simulink model "FingerEAERCtrl"  (R2012b)
settings: Solver=ode3  StartTime=0.0  StopTime=inf  FixedStep=.001  RelTol=1e-3
PreLoadFcn:
  | settupFilter;
InitFcn:
  | settupFilter;
values from neighbouring files (symbols this model uses):
  x0low = (eye(size(Alow))-Alow)\Blow*0    [settupFilter.m]
undefined symbols (not defined in the file or in its folder): Alow, Blow, Clow, Dlow
libraries: xpcnilib x4, xpclib x4, simulink x2
(part 2 of 2)

== system FingerEAERCtrl/trajectory calculator/mode 4: sub init no return/rt minimum jerk trajectory1/params buffer1 ==
  pDes_ : Inport
  tHit_ : Inport  Port=2
  maxDur : Inport  Port=3
  t : Inport  Port=4
  Trigger : TriggerPort  PortDimensions=1
  Memory : Memory  InheritSampleTime=on
  Memory1 : Memory  InheritSampleTime=on
  buffer the trajectory params : MATLAB Function  TreatAsAtomicUnit=on
  pDes : Outport
  tHit : Outport  Port=2
  dur : Outport  Port=3
  wires:
  pDes_/1 -> buffer the trajectory params/1(pDes_)
  buffer the trajectory params/1(pDes) -> pDes/1
  buffer the trajectory params/2(tHit) -> Memory/1, tHit/1
  tHit_/1 -> buffer the trajectory params/2(tHit_)
  t/1 -> buffer the trajectory params/4(t)
  maxDur/1 -> buffer the trajectory params/3(maxDur)
  buffer the trajectory params/3(dur) -> Memory1/1, dur/1
  Memory/1 -> buffer the trajectory params/5(lastHit)
  Memory1/1 -> buffer the trajectory params/6(lastDur)

== system FingerEAERCtrl/trajectory calculator/mode 4: sub init no return/rt minimum jerk trajectory1/saveTrialStartTime ==
  t : Inport
  Trigger : TriggerPort  PortDimensions=1
  save the trial start time : MATLAB Function  TreatAsAtomicUnit=on
  trialStartTime : Outport
  wires:
  t/1 -> save the trial start time/1(t)
  save the trial start time/1(trialStartTime) -> trialStartTime/1

== system FingerEAERCtrl/trajectory calculator/mode 4: sub init no return/rt minimum jerk trajectory1/timeToTrigger ==
  note: This block (triggered by passing the force threshold / success in the movement initiation)
      | checks to make sure that it wasn't a subsequent trigger, and if it wasn't, passes the time
      | from the trial start to the time of the trigger event (time to meet the force threshold) as feedback
  t : Inport
  trialStart : Inport  Port=2
  Trigger : TriggerPort  PortDimensions=1
  Memory : Memory  InheritSampleTime=on
  Memory1 : Memory  InheritSampleTime=on
  save the trigger time : MATLAB Function  TreatAsAtomicUnit=on
  triggerTime : Outport
  wires:
  t/1 -> save the trigger time/2(t)
  trialStart/1 -> save the trigger time/3(trialStart)
  save the trigger time/2(lastStartT) -> Memory/1
  Memory/1 -> save the trigger time/4(lastTrialStart)
  save the trigger time/1(triggerTime) -> Memory1/1, triggerTime/1
  Memory1/1 -> save the trigger time/1(lastTriggerTime)

== system FingerEAERCtrl/trajectory calculator/mode 4: sub init no return/rt minimum jerk trajectory2/detect new trajectory ==
  note: detects when tDes is changed, and trips the trigger
  tDes : Inport
  MATLAB Function1 : MATLAB Function  TreatAsAtomicUnit=on
  Memory2 : Memory
  change : Outport
  wires:
  tDes/1 -> MATLAB Function1/1(tDes)
  MATLAB Function1/1(change) -> change/1
  MATLAB Function1/2(tDesOut) -> Memory2/1
  Memory2/1 -> MATLAB Function1/2(tDesLast)

== system FingerEAERCtrl/trajectory calculator/mode 4: sub init no return/rt minimum jerk trajectory2/force buffer ==
  force_ : Inport
  Trigger : TriggerPort  PortDimensions=1
  buffer the initial force value : MATLAB Function  TreatAsAtomicUnit=on
  force : Outport
  wires:
  force_/1 -> buffer the initial force value/1(force_)
  buffer the initial force value/1(force) -> force/1

== system FingerEAERCtrl/trajectory calculator/mode 4: sub init no return/rt minimum jerk trajectory2/params buffer1 ==
  pDes_ : Inport
  tHit_ : Inport  Port=2
  maxDur : Inport  Port=3
  t : Inport  Port=4
  Trigger : TriggerPort  PortDimensions=1
  Memory : Memory  InheritSampleTime=on
  Memory1 : Memory  InheritSampleTime=on
  buffer the trajectory params : MATLAB Function  TreatAsAtomicUnit=on
  pDes : Outport
  tHit : Outport  Port=2
  dur : Outport  Port=3
  wires:
  pDes_/1 -> buffer the trajectory params/1(pDes_)
  buffer the trajectory params/1(pDes) -> pDes/1
  buffer the trajectory params/2(tHit) -> Memory/1, tHit/1
  tHit_/1 -> buffer the trajectory params/2(tHit_)
  t/1 -> buffer the trajectory params/4(t)
  maxDur/1 -> buffer the trajectory params/3(maxDur)
  buffer the trajectory params/3(dur) -> Memory1/1, dur/1
  Memory/1 -> buffer the trajectory params/5(lastHit)
  Memory1/1 -> buffer the trajectory params/6(lastDur)

== system FingerEAERCtrl/trajectory calculator/mode 4: sub init no return/rt minimum jerk trajectory2/saveTrialStartTime ==
  t : Inport
  Trigger : TriggerPort  PortDimensions=1
  save the trial start time : MATLAB Function  TreatAsAtomicUnit=on
  trialStartTime : Outport
  wires:
  t/1 -> save the trial start time/1(t)
  save the trial start time/1(trialStartTime) -> trialStartTime/1

== system FingerEAERCtrl/trajectory calculator/mode 4: sub init no return/rt minimum jerk trajectory2/timeToTrigger ==
  note: This block (triggered by passing the force threshold / success in the movement initiation)
      | checks to make sure that it wasn't a subsequent trigger, and if it wasn't, passes the time
      | from the trial start to the time of the trigger event (time to meet the force threshold) as feedback
  t : Inport
  trialStart : Inport  Port=2
  Trigger : TriggerPort  PortDimensions=1
  Memory : Memory  InheritSampleTime=on
  Memory1 : Memory  InheritSampleTime=on
  save the trigger time : MATLAB Function  TreatAsAtomicUnit=on
  triggerTime : Outport
  wires:
  t/1 -> save the trigger time/2(t)
  trialStart/1 -> save the trigger time/3(trialStart)
  save the trigger time/2(lastStartT) -> Memory/1
  Memory/1 -> save the trigger time/4(lastTrialStart)
  save the trigger time/1(triggerTime) -> Memory1/1, triggerTime/1
  Memory1/1 -> save the trigger time/1(lastTriggerTime)

== matlab function FingerEAERCtrl/trajectory calculator/mode 1: sub-init/rt minimum jerk trajectory calc/detect movement onset ==
  data: pos input; vel input; V_THRESH input; tDes input; update output; t input; pTraj input; maxDur input
% this function will detect when the subject startes to move. As soon as
% the subject's velocity reaches a certain threshold, get the distance to
% the target and the start time
function update = checkUpdate(pos, vel, V_THRESH, tDes, t, pTraj, maxDur)
%#codegen
update = 0;
if ((vel > V_THRESH) && (t < tDes) && (pTraj == 0))
    %% add another condition to make sure that the robot does not try to move super fast
    if ((abs(tDes - t) > .15) && (abs(tDes - t) < maxDur))
        update = 1;
    end    
end

== matlab function FingerEAERCtrl/controller/controller ==
  data: stateDes input; Forces output; state input; Kp input; Kd input
function Forces = pdCtrl(stateDes, state, Kp, Kd)
%#codegen
pDes = [stateDes(1); stateDes(4)];
vDes = [stateDes(2); stateDes(5)];

pos = [state(1); state(3)];
vel = [state(2); state(4)];

error = pDes - pos;
errorDot = vDes - vel;

Forces = error.*Kp + errorDot.*Kd;

== matlab function FingerEAERCtrl/trajectory calculator/mode 1: sub-init/rt minimum jerk trajectory calc/params buffer/buffer the trajectory params ==
  data: pDes output; tHit output; pDes_ input; tHit_ input; t input; dur output
function [pDes, tHit, dur] = bufferParams(pDes_, tHit_, t)
%#codegen
pDes = pDes_;
tHit = tHit_;
dur = tHit_ - t;
% Ro = abs(pDes - pos)
% to = t
% tr = tDes - to

== matlab function FingerEAERCtrl/trajectory calculator/mode 1: sub-init/rt minimum jerk trajectory calc/MATLAB Function ==
  data: Pd input; th input; dur input; des output; t input
% th is the hit time
% Pd id the final destination
% t is the current time
% dur is the duration 
function des = trajCalc(Pd, th, dur, t)
%#codegen
startT = th - dur;  % number of miliseconds until the hit time
returnT = th + dur;  % return time

if t > startT && t<=th
T=t-(startT);
des=[(10*Pd*T^3)/dur^3 - (15*Pd*T^4)/dur^4 + (6*Pd*T^5)/dur^5;...
(30*Pd*T^2)/dur^3 - (60*Pd*T^3)/dur^4 + (30*Pd*T^4)/dur^5;...
(120*Pd*T^3)/dur^5 - (180*Pd*T^2)/dur^4 + (60*Pd*T)/dur^3];
elseif th<t && t<returnT
T=t-th;
des=[Pd - (10*Pd*T^3)/dur^3 + (15*Pd*T^4)/dur^4 - (6*Pd*T^5)/dur^5;...
(60*Pd*T^3)/dur^4 - (30*Pd*T^2)/dur^3 - (30*Pd*T^4)/dur^5;...
(180*Pd*T^2)/dur^4 - (120*Pd*T^3)/dur^5 - (60*Pd*T)/dur^3];
else
des=[0;0;0];
end

== matlab function FingerEAERCtrl/trajectory calculator/mode 3: auto init no return/rt minimum jerk trajectory/MATLAB Function ==
  data: Pd input; th input; dur input; des output; t input; Phold_ input; Phold output; state_ input; state output
% th is the hit time
% Pd id the final destination
% t is the current time
% dur is the duration 
function [des, Phold, state] = trajCalc(Pd, th, dur, t, Phold_, state_)
startT = th - dur;  % number of miliseconds until the hit time

Pr = Pd - Phold_;
Phold = Phold_;
state = state_;
switch state_
    case 0
        des = [Phold_; 0; 0];
        if (t > startT); state = 1; end
    case 1
        T=t-(startT);
        des=[(10*Pr*T^3)/dur^3 - (15*Pr*T^4)/dur^4 + (6*Pr*T^5)/dur^5 + Phold_;...
        (30*Pr*T^2)/dur^3 - (60*Pr*T^3)/dur^4 + (30*Pr*T^4)/dur^5;...
        (120*Pr*T^3)/dur^5 - (180*Pr*T^2)/dur^4 + (60*Pr*T)/dur^3];
        if (t > th); state = 2; end
    case 2
        Phold = Pd;
        des = [Pd; 0; 0];
        state = 3;
    case 3
        des = [Phold_; 0; 0];
        if (t < startT); state = 0; end
    otherwise
        state = 0;
        Phold = 0;
        des = [Phold_; 0; 0];
end

== matlab function FingerEAERCtrl/trajectory calculator/mode 3: auto init no return/rt minimum jerk trajectory/detect change/MATLAB Function1 ==
  data: pDes input; change output; pDes_ input
function change = detectChange(pDes, pDes_)
%#codegen
change = 0
diffS = pDes - pDes_;
if (diffS > 0) && (pDes_ == 0)
    change = 1;
end

== matlab function FingerEAERCtrl/trajectory calculator/mode 3: auto init no return/rt minimum jerk trajectory/params buffer/buffer the trajectory params ==
  data: pDes output; tHit output; pDes_ input; tHit_ input
function [pDes, tHit] = bufferParams(pDes_, tHit_)
%#codegen
pDes = pDes_;
tHit = tHit_;
% Ro = abs(pDes - pos)
% to = t
% tr = tDes - to

== matlab function FingerEAERCtrl/controller/gain transition/gainramp ==
  data: val output; tr input; valD input; state1 output; state input
% state contains [valD_,val_,Ro_,t_]
function [val,state1] = fcn(tr,valD,state)
%#eml

% first we need to check if they have changed the desired Value
if ~ (valD == state(1))
    state(1) = valD;
    state(4) = 0;
    state(3) = state(1) - state(2);
end

t = state(4);
Ro = state(3);

if ((t <= tr) && (tr~=0))
    Rd = Ro - Ro*(10*(t)^3/(tr)^3 - 15*(t)^4/(tr)^4 + 6*(t)^5/(tr)^5);
else
    Rd = 0;
end

val = state(1) - Rd;
state(2) = val;
state(4) = t + .001;
state1 = state;

== matlab function FingerEAERCtrl/Robot/get offsets/MATLAB Function ==
  data: enc1_ input; encoder1 output; enc2_ input; time input; summedVals_ input; nSamples_ input; encoder2 output; summedVals output; nSamples output
%% remove the position offset that comes from using the encoders for
% feedback
%%
function [encoder1, encoder2, summedVals, nSamples] = getOffset(enc1_, enc2_, time, summedVals_, nSamples_)
%#codegen
summedVals = summedVals_;
if (time > 2) && (time < 3)
    summedVals(1) = summedVals_(1) + enc1_;
    summedVals(2) = summedVals_(2) + enc2_;
    nSamples = nSamples_ + 1;
    encoder1 = 0;
    encoder2 = 0;
elseif (time >=3)
    summedVals = summedVals_;
    nSamples = nSamples_;
    encoder1 = enc1_ - summedVals(1)/nSamples;
    encoder2 = enc2_ - summedVals(2)/nSamples;
else (time <= 2)
    summedVals = summedVals_;
    nSamples = nSamples_;
    encoder1 = 0;
    encoder2 = 0;
end

== matlab function FingerEAERCtrl/controller/initial ramp/MATLAB Function ==
  data: ctrlForce input; Force output; rampForce input; time input
function Force = blendForces(ctrlForce, rampForce, time)
%#codegen
transitionTime = 5.0;
ctrlW = 1 ./ (1 + exp(-8*(time - transitionTime)) );
Force = ctrlW*ctrlForce + (1 - ctrlW)*rampForce;

== matlab function FingerEAERCtrl/Robot/account for handedness/MATLAB Function ==
  data: input1 input; output1 output; input2 input; leftyMode input; output2 output
% encoder 1 and output 1 relate to the blue mechanism
% encoder 2, output 2 and accel 2 relate to the gold mechanism
% in right hand mode, we want the gold mechanism to control the index finger
% in left hand mode, we want the blue mechanism to control the index finger

% we wallways want the index finger to be finger 1

function [output1, output2] = fcn(input1, input2, leftyMode)
%#codegen
if leftyMode == 1
    output1 = input1;
    output2 = input2;
else
    output1 = input2;
    output2 = input1;
end

== matlab function FingerEAERCtrl/Robot/account for handedness1/MATLAB Function ==
  data: input1 input; output1 output; input2 input; leftyMode input; output2 output
% encoder 1 and output 1 relate to the blue mechanism
% encoder 2, output 2 and accel 2 relate to the gold mechanism
% in right hand mode, we want the gold mechanism to control the index finger
% in left hand mode, we want the blue mechanism to control the index finger

% we wallways want the index finger to be finger 1

function [output1, output2] = fcn(input1, input2, leftyMode)
%#codegen
if leftyMode == 1
    output1 = input1;
    output2 = input2;
else
    output1 = input2;
    output2 = input1;
end

== matlab function FingerEAERCtrl/Robot/account for handedness2/MATLAB Function ==
  data: input1 input; output1 output; input2 input; leftyMode input; output2 output
% encoder 1 and output 1 relate to the blue mechanism
% encoder 2, output 2 and accel 2 relate to the gold mechanism
% in right hand mode, we want the gold mechanism to control the index finger
% in left hand mode, we want the blue mechanism to control the index finger

% we wallways want the index finger to be finger 1

function [output1, output2] = fcn(input1, input2, leftyMode)
%#codegen
if leftyMode == 1
    output1 = input1;
    output2 = input2;
else
    output1 = input2;
    output2 = input1;
end

== matlab function FingerEAERCtrl/parameters/gain transition/gainramp ==
  data: val output; tr input; valD input; state1 output; state input
% state contains [valD_,val_,Ro_,t_]
function [val,state1] = fcn(tr,valD,state)
%#eml

% first we need to check if they have changed the desired Value
if ~ (valD == state(1))
    state(1) = valD;
    state(4) = 0;
    state(3) = state(1) - state(2);
end

t = state(4);
Ro = state(3);

if ((t <= tr) && (tr~=0))
    Rd = Ro - Ro*(10*(t)^3/(tr)^3 - 15*(t)^4/(tr)^4 + 6*(t)^5/(tr)^5);
else
    Rd = 0;
end

val = state(1) - Rd;
state(2) = val;
state(4) = t + .001;
state1 = state;

== matlab function FingerEAERCtrl/parameters/gain transition1/gainramp ==
  data: val output; tr input; valD input; state1 output; state input
% state contains [valD_,val_,Ro_,t_]
function [val,state1] = fcn(tr,valD,state)
%#eml

% first we need to check if they have changed the desired Value
if ~ (valD == state(1))
    state(1) = valD;
    state(4) = 0;
    state(3) = state(1) - state(2);
end

t = state(4);
Ro = state(3);

if ((t <= tr) && (tr~=0))
    Rd = Ro - Ro*(10*(t)^3/(tr)^3 - 15*(t)^4/(tr)^4 + 6*(t)^5/(tr)^5);
else
    Rd = 0;
end

val = state(1) - Rd;
state(2) = val;
state(4) = t + .001;
state1 = state;

== matlab function FingerEAERCtrl/parameters/gain transition2/gainramp ==
  data: val output; tr input; valD input; state1 output; state input
% state contains [valD_,val_,Ro_,t_]
function [val,state1] = fcn(tr,valD,state)
%#eml

% first we need to check if they have changed the desired Value
if ~ (valD == state(1))
    state(1) = valD;
    state(4) = 0;
    state(3) = state(1) - state(2);
end

t = state(4);
Ro = state(3);

if ((t <= tr) && (tr~=0))
    Rd = Ro - Ro*(10*(t)^3/(tr)^3 - 15*(t)^4/(tr)^4 + 6*(t)^5/(tr)^5);
else
    Rd = 0;
end

val = state(1) - Rd;
state(2) = val;
state(4) = t + .001;
state1 = state;

== matlab function FingerEAERCtrl/parameters/gain transition3/gainramp ==
  data: val output; tr input; valD input; state1 output; state input
% state contains [valD_,val_,Ro_,t_]
function [val,state1] = fcn(tr,valD,state)
%#eml

% first we need to check if they have changed the desired Value
if ~ (valD == state(1))
    state(1) = valD;
    state(4) = 0;
    state(3) = state(1) - state(2);
end

t = state(4);
Ro = state(3);

if ((t <= tr) && (tr~=0))
    Rd = Ro - Ro*(10*(t)^3/(tr)^3 - 15*(t)^4/(tr)^4 + 6*(t)^5/(tr)^5);
else
    Rd = 0;
end

val = state(1) - Rd;
state(2) = val;
state(4) = t + .001;
state1 = state;

== matlab function FingerEAERCtrl/trajectory calculator/mode 3: auto init no return/rt minimum jerk trajectory1/MATLAB Function ==
  data: Pd input; th input; dur input; des output; t input; Phold_ input; Phold output; state_ input; state output
% th is the hit time
% Pd id the final destination
% t is the current time
% dur is the duration 
function [des, Phold, state] = trajCalc(Pd, th, dur, t, Phold_, state_)
startT = th - dur;  % number of miliseconds until the hit time

Pr = Pd - Phold_;
Phold = Phold_;
state = state_;
switch state_
    case 0
        des = [Phold_; 0; 0];
        if (t > startT); state = 1; end
    case 1
        T=t-(startT);
        des=[(10*Pr*T^3)/dur^3 - (15*Pr*T^4)/dur^4 + (6*Pr*T^5)/dur^5 + Phold_;...
        (30*Pr*T^2)/dur^3 - (60*Pr*T^3)/dur^4 + (30*Pr*T^4)/dur^5;...
        (120*Pr*T^3)/dur^5 - (180*Pr*T^2)/dur^4 + (60*Pr*T)/dur^3];
        if (t > th); state = 2; end
    case 2
        Phold = Pd;
        des = [Pd; 0; 0];
        state = 3;
    case 3
        des = [Phold_; 0; 0];
        if (t < startT); state = 0; end
    otherwise
        state = 0;
        Phold = 0;
        des = [Phold_; 0; 0];
end

== matlab function FingerEAERCtrl/trajectory calculator/mode 1: sub-init/rt minimum jerk trajectory calc1/MATLAB Function ==
  data: Pd input; th input; dur input; des output; t input
% th is the hit time
% Pd id the final destination
% t is the current time
% dur is the duration 
function des = trajCalc(Pd, th, dur, t)
%#codegen
startT = th - dur;  % number of miliseconds until the hit time
returnT = th + dur;  % return time

if t > startT && t<=th
T=t-(startT);
des=[(10*Pd*T^3)/dur^3 - (15*Pd*T^4)/dur^4 + (6*Pd*T^5)/dur^5;...
(30*Pd*T^2)/dur^3 - (60*Pd*T^3)/dur^4 + (30*Pd*T^4)/dur^5;...
(120*Pd*T^3)/dur^5 - (180*Pd*T^2)/dur^4 + (60*Pd*T)/dur^3];
elseif th<t && t<returnT
T=t-th;
des=[Pd - (10*Pd*T^3)/dur^3 + (15*Pd*T^4)/dur^4 - (6*Pd*T^5)/dur^5;...
(60*Pd*T^3)/dur^4 - (30*Pd*T^2)/dur^3 - (30*Pd*T^4)/dur^5;...
(180*Pd*T^2)/dur^4 - (120*Pd*T^3)/dur^5 - (60*Pd*T)/dur^3];
else
des=[0;0;0];
end

== matlab function FingerEAERCtrl/trajectory calculator/mode 3: auto init no return/rt minimum jerk trajectory1/detect change/MATLAB Function1 ==
  data: pDes input; change output; pDes_ input
function change = detectChange(pDes, pDes_)
%#codegen
change = 0
diffS = pDes - pDes_;
if (diffS > 0) && (pDes_ == 0)
    change = 1;
end

== matlab function FingerEAERCtrl/trajectory calculator/mode 3: auto init no return/rt minimum jerk trajectory1/params buffer/buffer the trajectory params ==
  data: pDes output; tHit output; pDes_ input; tHit_ input
function [pDes, tHit] = bufferParams(pDes_, tHit_)
%#codegen
pDes = pDes_;
tHit = tHit_;
% Ro = abs(pDes - pos)
% to = t
% tr = tDes - to

== matlab function FingerEAERCtrl/trajectory calculator/mode 1: sub-init/rt minimum jerk trajectory calc1/detect force onset ==
  data: force input; F_THRESH input; tDes input; update output; t input; pTraj input; maxDur input
% this function will detect when the subject startes to move. As soon as
% the subject's velocity reaches a certain threshold, get the distance to
% the target and the start time
function update = checkUpdate(force, F_THRESH, tDes, t, pTraj, maxDur)
%#codegen
update = 0;
if ((force > F_THRESH) && (t < tDes) && (pTraj == 0))
    %% add another condition to make sure that the robot does not try to move super fast
    if ((abs(tDes - t) > .15) && (abs(tDes - t) < maxDur))
        update = 1;
    end    
end

== matlab function FingerEAERCtrl/trajectory calculator/mode 4: sub init no return/rt minimum jerk trajectory1/saveTrialStartTime/save the trial start time ==
  data: trialStartTime output; t input
function trialStartTime = getTrialStartTime(t)
trialStartTime = t;
end

== matlab function FingerEAERCtrl/trajectory calculator/mode 1: sub-init/rt minimum jerk trajectory calc1/detect movement onset ==
  data: pos input; vel input; V_THRESH input; tDes input; update output; t input; pTraj input; maxDur input
% this function will detect when the subject startes to move. As soon as
% the subject's velocity reaches a certain threshold, get the distance to
% the target and the start time
function update = checkUpdate(pos, vel, V_THRESH, tDes, t, pTraj, maxDur)
%#codegen
update = 0;
if ((vel > V_THRESH) && (t < tDes) && (pTraj == 0))
    %% add another condition to make sure that the robot does not try to move super fast
    if ((abs(tDes - t) > .15) && (abs(tDes - t) < maxDur))
        update = 1;
    end    
end

== matlab function FingerEAERCtrl/trajectory calculator/mode 1: sub-init/rt minimum jerk trajectory calc1/params buffer/buffer the trajectory params ==
  data: pDes output; tHit output; pDes_ input; tHit_ input; t input; dur output
function [pDes, tHit, dur] = bufferParams(pDes_, tHit_, t)
%#codegen
pDes = pDes_;
tHit = tHit_;
dur = tHit_ - t;
% Ro = abs(pDes - pos)
% to = t
% tr = tDes - to

== matlab function FingerEAERCtrl/Robot/account for handedness force/MATLAB Function ==
  data: inp1 input; output output; leftyMode input
% channel1 - gold tip
% channel2 - blue tip
% channel3 - gold base
% channel4 - blue base
% we wallways want the index finger to be finger 1

function output = fcn(inp1, leftyMode)
%#codegen

if leftyMode == 1
    output = [inp1(4); inp1(2); inp1(3); inp1(1); inp1(5)];
else
    output = [inp1(3); inp1(1); inp1(4); inp1(2); inp1(5)];
    %output = [inp1(3,1); inp1(4,2); inp1(5)];
end

== matlab function FingerEAERCtrl/trajectory calculator/mode 2: auto initiated/rt minimum jerk trajectory1/MATLAB Function ==
  data: Pd input; Pstart input; th input; dur input; des output; t input
% th is the hit time
% Pd id the final destination
% t is the current time
% dur is the duration 
function des = trajCalc(Pd, Pstart, th, dur, t)
%#codegen
startT = th - dur;  % number of miliseconds until the hit time
returnT = th + dur;  % return time

Prel = Pd - Pstart;

if t > startT && t<=th
T=t-(startT);
des=[(10*Prel*T^3)/dur^3 - (15*Prel*T^4)/dur^4 + (6*Prel*T^5)/dur^5 + Pstart;...
(30*Prel*T^2)/dur^3 - (60*Prel*T^3)/dur^4 + (30*Prel*T^4)/dur^5;...
(120*Prel*T^3)/dur^5 - (180*Prel*T^2)/dur^4 + (60*Prel*T)/dur^3];
elseif th<t && t<returnT
T=t-th;
des=[Pd - (10*Pd*T^3)/dur^3 + (15*Pd*T^4)/dur^4 - (6*Pd*T^5)/dur^5;...
(60*Pd*T^3)/dur^4 - (30*Pd*T^2)/dur^3 - (30*Pd*T^4)/dur^5;...
(180*Pd*T^2)/dur^4 - (120*Pd*T^3)/dur^5 - (60*Pd*T)/dur^3];
else
des=[0;0;0];
end

if des(2) < 0
    des(2) = 0;
end

== matlab function FingerEAERCtrl/trajectory calculator/mode 2: auto initiated/rt minimum jerk trajectory1/detect change/MATLAB Function1 ==
  data: pDes input; change output; pDes_ input
function change = detectChange(pDes, pDes_)
%#codegen
change = 0
diffS = pDes - pDes_;
if (diffS > 0) && (pDes_ == 0)
    change = 1;
end

== matlab function FingerEAERCtrl/trajectory calculator/mode 2: auto initiated/rt minimum jerk trajectory1/params buffer/buffer the trajectory params ==
  data: pDes output; pos output; tHit output; pDes_ input; pos_ input; tHit_ input; t input
function [pDes, pos, tHit] = bufferParams(pDes_, pos_, tHit_, t)
%#codegen
pDes = pDes_;
pos = pos_;
tHit = tHit_;
% Ro = abs(pDes - pos)
% to = t
% tr = tDes - to

== matlab function FingerEAERCtrl/controller/make chirp/MATLAB Function ==
  data: now input; f1 output; trigger input; wiggleAmp input; tStart input; f2 output; tStart_ output; fNum_ output; fNum input
function [f1, f2, tStart_, fNum_] = generateWiggle(now, trigger, wiggleAmp, tStart, fNum)
%#codegen
tStart_ = tStart;
fNum_ = fNum;
if trigger == 1
    tStart_ = now;
    fNum_ = trigger;
elseif trigger == 2
    tStart_ = now;
    fNum_ = trigger;
end

t = now - tStart;

tmax = 10;
fmax = 6;
fmin = .1;
k = (fmax/fmin)*(1/tmax);
f = fmin*k*t;

force = wiggleAmp*sin(2*pi*f*t);
if t > tmax
    force = 0;
end

if fNum == 1
    f1 = force;
    f2 = 0;
elseif fNum == 2
    f1 = 0;
    f2 = force;
else
    f1 = 0;
    f2 = 0;
end

== matlab function FingerEAERCtrl/controller/make chirp/MATLAB Function1 ==
  data: trigger input; pulse output; oldTrigger input; oldTrigger_ output
function [pulse, oldTrigger_] = detectForceTrigger(trigger, oldTrigger)
%#codegen

pulse = 0;
oldTrigger_ = oldTrigger;
if trigger ~= oldTrigger
    pulse = trigger;
    oldTrigger_ = trigger;
end

== matlab function FingerEAERCtrl/trajectory calculator/mode 4: sub init no return/rt minimum jerk trajectory1/timeToTrigger/save the trigger time ==
  data: lastTriggerTime input; triggerTime output; lastStartT output; t input; trialStart input; lastTrialStart input
function [triggerTime,lastStartT] = getTriggerTime(lastTriggerTime, t, trialStart, lastTrialStart)
% make sure this is not a subsequent trigger (we don't want those to
% update the time to trigger time value - we only want the first one)
if trialStart ~= lastTrialStart
    triggerTime = t-trialStart;    
else
    triggerTime = lastTriggerTime;
end

% update the trial start time regardless
lastStartT = trialStart;

end

== matlab function FingerEAERCtrl/trajectory calculator/mode 4: sub init no return/rt minimum jerk trajectory2/MATLAB Function ==
  data: Pd input; th input; dur input; des output; t input; Phold_ input; Phold output; state_ input; state output
% th is the hit time
% Pd id the final destination
% t is the current time
% dur is the duration 
function [des, Phold, state] = trajCalc(Pd, th, dur, t, Phold_, state_)
startT = th - dur;  % number of miliseconds until the hit time

Pr = Pd - Phold_;
Phold = Phold_;
state = state_;
switch state_
    case 0
        des = [Phold_; 0; 0];
        if (t > startT); state = 1; end
    case 1
        T=t-(startT);
        des=[(10*Pr*T^3)/dur^3 - (15*Pr*T^4)/dur^4 + (6*Pr*T^5)/dur^5 + Phold_;...
        (30*Pr*T^2)/dur^3 - (60*Pr*T^3)/dur^4 + (30*Pr*T^4)/dur^5;...
        (120*Pr*T^3)/dur^5 - (180*Pr*T^2)/dur^4 + (60*Pr*T)/dur^3];
        if (t > th); state = 2; end
    case 2
        Phold = Pd;
        des = [Pd; 0; 0];
        state = 3;
    case 3
        des = [Phold_; 0; 0];
        if (t < startT); state = 0; end
    otherwise
        state = 0;
        Phold = 0;
        des = [Phold_; 0; 0];
end

== matlab function FingerEAERCtrl/trajectory calculator/mode 2: auto initiated/rt minimum jerk trajectory/MATLAB Function ==
  data: Pd input; Pstart input; th input; dur input; des output; t input
% th is the hit time
% Pd id the final destination
% t is the current time
% dur is the duration 
function des = trajCalc(Pd, Pstart, th, dur, t)
%#codegen
startT = th - dur;  % number of miliseconds until the hit time
returnT = th + dur;  % return time

Prel = Pd - Pstart;

if t > startT && t<=th
T=t-(startT);
des=[(10*Prel*T^3)/dur^3 - (15*Prel*T^4)/dur^4 + (6*Prel*T^5)/dur^5 + Pstart;...
(30*Prel*T^2)/dur^3 - (60*Prel*T^3)/dur^4 + (30*Prel*T^4)/dur^5;...
(120*Prel*T^3)/dur^5 - (180*Prel*T^2)/dur^4 + (60*Prel*T)/dur^3];
elseif th<t && t<returnT
T=t-th;
des=[Pd - (10*Pd*T^3)/dur^3 + (15*Pd*T^4)/dur^4 - (6*Pd*T^5)/dur^5;...
(60*Pd*T^3)/dur^4 - (30*Pd*T^2)/dur^3 - (30*Pd*T^4)/dur^5;...
(180*Pd*T^2)/dur^4 - (120*Pd*T^3)/dur^5 - (60*Pd*T)/dur^3];
else
des=[0;0;0];
end

if des(2) < 0
    des(2) = 0;
end

== matlab function FingerEAERCtrl/trajectory calculator/mode 4: sub init no return/rt minimum jerk trajectory2/detect force onset1 ==
  data: Pdes input; force input; F_THRESH input; tDes input; update output; t input; f0 input; maxDur input
% this function will detect when the subject startes to move. As soon as
% the subject's velocity reaches a certain threshold, get the distance to
% the target and the start time
function update = checkUpdate(Pdes, force, F_THRESH, tDes, t, f0, maxDur)
update = 0;

% change force to a difference based on a baseline value
force = force-f0;

% reverse force requirement if in extension
if Pdes < 0.5
    force = -force;
end

% check for threshold within time window
if (force > F_THRESH) && (t < tDes) && ((tDes-t) < maxDur)
    update = 1;
end
end

== matlab function FingerEAERCtrl/trajectory calculator/mode 2: auto initiated/rt minimum jerk trajectory/detect change/MATLAB Function1 ==
  data: pDes input; change output; pDes_ input
function change = detectChange(pDes, pDes_)
%#codegen
change = 0
diffS = pDes - pDes_;
if (diffS > 0) && (pDes_ == 0)
    change = 1;
end

== matlab function FingerEAERCtrl/trajectory calculator/mode 4: sub init no return/rt minimum jerk trajectory2/detect movement onset1 ==
  data: vel input; V_THRESH input; tDes input; update output; t input; maxDur input
% this function will detect when the subject startes to move. As soon as
% the subject's velocity reaches a certain threshold, get the distance to
% the target and the start time
function update = checkUpdate(vel, V_THRESH, tDes, t, maxDur)
%#codegen
update = 0;

vel = abs(vel);
if (vel > V_THRESH) && (t < tDes) &&((tDes-t) < maxDur)
    update = 1;
end
end

== matlab function FingerEAERCtrl/trajectory calculator/mode 2: auto initiated/rt minimum jerk trajectory/params buffer/buffer the trajectory params ==
  data: pDes output; pos output; tHit output; pDes_ input; pos_ input; tHit_ input; t input
function [pDes, pos, tHit] = bufferParams(pDes_, pos_, tHit_, t)
%#codegen
pDes = pDes_;
pos = pos_;
tHit = tHit_;
% Ro = abs(pDes - pos)
% to = t
% tr = tDes - to

== matlab function FingerEAERCtrl/trajectory calculator/mode 4: sub init no return/rt minimum jerk trajectory2/detect new trajectory/MATLAB Function1 ==
  data: tDes input; change output; tDesLast input; tDesOut output
function [change, tDesOut] = detectChange(tDes, tDesLast)
if (tDes~=tDesLast) 
    change = 1;
else
    change=0;
end
tDesOut = tDes;
end

== matlab function FingerEAERCtrl/trajectory calculator/mode 4: sub init no return/rt minimum jerk trajectory2/force buffer/buffer the initial force value ==
  data: force output; force_ input
function force = forceBuffer(force_)
force = force_;
end

== matlab function FingerEAERCtrl/trajectory calculator/mode 4: sub init no return/rt minimum jerk trajectory2/params buffer1/buffer the trajectory params ==
  data: pDes output; tHit output; pDes_ input; tHit_ input; maxDur input; dur output; t input; lastHit input; lastDur input
function [pDes, tHit, dur] = bufferParams(pDes_, tHit_, maxDur, t, lastHit, lastDur)
%#codegen
%% %% make sure we have a new hit time before passing the parameters
if (tHit_ == lastHit)    
    pDes = pDes_;
    tHit = lastHit;
    dur = lastDur;
    return
end
    
%% %% set new movement completeion parameters %%%%
pDes = pDes_;
tHit = tHit_;

%% %% calculate movement duration %%%%
minDur = maxDur/2;
time_left = abs(tHit_-t);

% this assumes that dur (which is the max dur) is greater than minDur
if (time_left > maxDur) 
    dur = maxDur;
elseif (time_left < maxDur) && (time_left > minDur)
    dur = time_left;
elseif (time_left < minDur)
    dur = minDur;
else
    dur = maxDur;
end

== matlab function FingerEAERCtrl/controller/viccosityAdder ==
  data: state input; stopPos input; KdVisc input; Forces output
function Forces = viscosity(state, stopPos, KdVisc)
%#codegen

pos = [state(1); state(3)];
vel = [state(2); state(4)];
Forces = [0.0; 0.0];
Forces(1) = -vel(1)*KdVisc(1);
Forces(2) = -vel(2)*KdVisc(2);

%% add in a software soft stop
% if the robot is close to the extreemes of it's range of motion, apply a
% viscous field to slow the robot down so that the user will not slam the
% mechanisms into the hard stops.

% softStopGain = .7;
maxSSGain = 2;
ssgM = (maxSSGain)/(1-stopPos);
b = -ssgM*stopPos;
softStopGain1 = ssgM*pos(1) + b;
softStopGain2 = ssgM*pos(2) + b;


if (pos(1) > stopPos) && (vel(1) > 0)
    Forces(1) = Forces(1) - vel(1)*softStopGain1;
end

if (pos(2) > stopPos) && (vel(2) > 0)
    Forces(2) = Forces(2) - vel(2)*softStopGain2;
end

== matlab function FingerEAERCtrl/parameters/gain transition4/gainramp ==
  data: val output; tr input; valD input; state1 output; state input
% state contains [valD_,val_,Ro_,t_]
function [val,state1] = fcn(tr,valD,state)
%#eml

% first we need to check if they have changed the desired Value
if ~ (valD == state(1))
    state(1) = valD;
    state(4) = 0;
    state(3) = state(1) - state(2);
end

t = state(4);
Ro = state(3);

if ((t <= tr) && (tr~=0))
    Rd = Ro - Ro*(10*(t)^3/(tr)^3 - 15*(t)^4/(tr)^4 + 6*(t)^5/(tr)^5);
else
    Rd = 0;
end

val = state(1) - Rd;
state(2) = val;
state(4) = t + .001;
state1 = state;

== matlab function FingerEAERCtrl/parameters/gain transition5/gainramp ==
  data: val output; tr input; valD input; state1 output; state input
% state contains [valD_,val_,Ro_,t_]
function [val,state1] = fcn(tr,valD,state)
%#eml

% first we need to check if they have changed the desired Value
if ~ (valD == state(1))
    state(1) = valD;
    state(4) = 0;
    state(3) = state(1) - state(2);
end

t = state(4);
Ro = state(3);

if ((t <= tr) && (tr~=0))
    Rd = Ro - Ro*(10*(t)^3/(tr)^3 - 15*(t)^4/(tr)^4 + 6*(t)^5/(tr)^5);
else
    Rd = 0;
end

val = state(1) - Rd;
state(2) = val;
state(4) = t + .001;
state1 = state;

== matlab function FingerEAERCtrl/controller/initial ramp/ramp ==
  data: tTime input; y output
function y = fcn(tTime)
%#codegen
slope = -0.8;
y = tTime*slope;

== matlab function FingerEAERCtrl/trajectory calculator/mode 1: sub-init/rt minimum jerk trajectory calc/detect force onset ==
  data: force input; F_THRESH input; tDes input; update output; t input; pTraj input; maxDur input
% this function will detect when the subject startes to move. As soon as
% the subject's velocity reaches a certain threshold, get the distance to
% the target and the start time
function update = checkUpdate(force, F_THRESH, tDes, t, pTraj, maxDur)
%#codegen
update = 0;
if ((force > F_THRESH) && (t < tDes) && (pTraj == 0))
    %% add another condition to make sure that the robot does not try to move super fast
    if ((abs(tDes - t) > .15) && (abs(tDes - t) < maxDur))
        update = 1;
    end    
end

== matlab function FingerEAERCtrl/trajectory calculator/mode 4: sub init no return/rt minimum jerk trajectory2/saveTrialStartTime/save the trial start time ==
  data: trialStartTime output; t input
function trialStartTime = getTrialStartTime(t)
trialStartTime = t;
end

== matlab function FingerEAERCtrl/trajectory calculator/mode 4: sub init no return/rt minimum jerk trajectory2/timeToTrigger/save the trigger time ==
  data: lastTriggerTime input; triggerTime output; lastStartT output; t input; trialStart input; lastTrialStart input
function [triggerTime,lastStartT] = getTriggerTime(lastTriggerTime, t, trialStart, lastTrialStart)
% make sure this is not a subsequent trigger (we don't want those to
% update the time to trigger time value - we only want the first one)
if trialStart ~= lastTrialStart
    triggerTime = t-trialStart;    
else
    triggerTime = lastTriggerTime;
end

% update the trial start time regardless
lastStartT = trialStart;

end

== matlab function FingerEAERCtrl/trajectory calculator/mode 4: sub init no return/rt minimum jerk trajectory1/MATLAB Function ==
  data: Pd input; th input; dur input; des output; t input; Phold_ input; Phold output; state_ input; state output
% th is the hit time
% Pd id the final destination
% t is the current time
% dur is the duration 
function [des, Phold, state] = trajCalc(Pd, th, dur, t, Phold_, state_)
startT = th - dur;  % number of miliseconds until the hit time

Pr = Pd - Phold_;
Phold = Phold_;
state = state_;
switch state_
    case 0
        des = [Phold_; 0; 0];
        if (t > startT); state = 1; end
    case 1
        T=t-(startT);
        des=[(10*Pr*T^3)/dur^3 - (15*Pr*T^4)/dur^4 + (6*Pr*T^5)/dur^5 + Phold_;...
        (30*Pr*T^2)/dur^3 - (60*Pr*T^3)/dur^4 + (30*Pr*T^4)/dur^5;...
        (120*Pr*T^3)/dur^5 - (180*Pr*T^2)/dur^4 + (60*Pr*T)/dur^3];
        if (t > th); state = 2; end
    case 2
        Phold = Pd;
        des = [Pd; 0; 0];
        state = 3;
    case 3
        des = [Phold_; 0; 0];
        if (t < startT); state = 0; end
    otherwise
        state = 0;
        Phold = 0;
        des = [Phold_; 0; 0];
end

== matlab function FingerEAERCtrl/trajectory calculator/mode 4: sub init no return/rt minimum jerk trajectory1/detect force onset1 ==
  data: Pdes input; force input; F_THRESH input; tDes input; update output; t input; f0 input; maxDur input
% this function will detect when the subject startes to move. As soon as
% the subject's velocity reaches a certain threshold, get the distance to
% the target and the start time
function update = checkUpdate(Pdes, force, F_THRESH, tDes, t, f0, maxDur)
update = 0;

% change force to a difference based on a baseline value
force = force-f0;

% reverse force requirement if in extension
if Pdes < 0.5
    force = -force;
end

% check for threshold within time window
if (force > F_THRESH) && (t < tDes) && ((tDes-t) < maxDur)
    update = 1;
end
end

== matlab function FingerEAERCtrl/trajectory calculator/mode 4: sub init no return/rt minimum jerk trajectory1/detect movement onset1 ==
  data: vel input; V_THRESH input; tDes input; update output; t input; maxDur input
% this function will detect when the subject startes to move. As soon as
% the subject's velocity reaches a certain threshold, get the distance to
% the target and the start time
function update = checkUpdate(vel, V_THRESH, tDes, t, maxDur)
%#codegen
update = 0;

vel = abs(vel);
if (vel > V_THRESH) && (t < tDes) &&((tDes-t) < maxDur)
    update = 1;
end
end

== matlab function FingerEAERCtrl/trajectory calculator/mode 4: sub init no return/rt minimum jerk trajectory1/detect new trajectory/MATLAB Function1 ==
  data: tDes input; change output; tDesLast input; tDesOut output
function [change, tDesOut] = detectChange(tDes, tDesLast)
if (tDes~=tDesLast) 
    change = 1;
else
    change=0;
end
tDesOut = tDes;
end

== matlab function FingerEAERCtrl/trajectory calculator/mode 4: sub init no return/rt minimum jerk trajectory1/force buffer/buffer the initial force value ==
  data: force output; force_ input
function force = forceBuffer(force_)
force = force_;
end

== matlab function FingerEAERCtrl/trajectory calculator/mode 4: sub init no return/rt minimum jerk trajectory1/params buffer1/buffer the trajectory params ==
  data: pDes output; tHit output; pDes_ input; tHit_ input; maxDur input; dur output; t input; lastHit input; lastDur input
function [pDes, tHit, dur] = bufferParams(pDes_, tHit_, maxDur, t, lastHit, lastDur)
%#codegen
%% %% make sure we have a new hit time before passing the parameters
if (tHit_ == lastHit)    
    pDes = pDes_;
    tHit = lastHit;
    dur = lastDur;
    return
end
    
%% %% set new movement completeion parameters %%%%
pDes = pDes_;
tHit = tHit_;

%% %% calculate movement duration %%%%
minDur = maxDur/2;
time_left = abs(tHit_-t);

% this assumes that dur (which is the max dur) is greater than minDur
if (time_left > maxDur) 
    dur = maxDur;
elseif (time_left < maxDur) && (time_left > minDur)
    dur = time_left;
elseif (time_left < minDur)
    dur = minDur;
else
    dur = maxDur;
end
